simulink model "controller_smp"  (R2021a)
settings: Solver=FixedStepAuto  StartTime=0.0  StopTime=10.0  FixedStep=1/10  RelTol=1e-3
settings Model: EnablePacing=on  PacingRate=3  Creator=DAUIN-Win10  LastModifiedBy=augus
settings DataIOCC: SaveOutput=off  SaveTime=off
settings GRTTargetCC: CombineOutputUpdateFcns=off  MatFileLogging=off

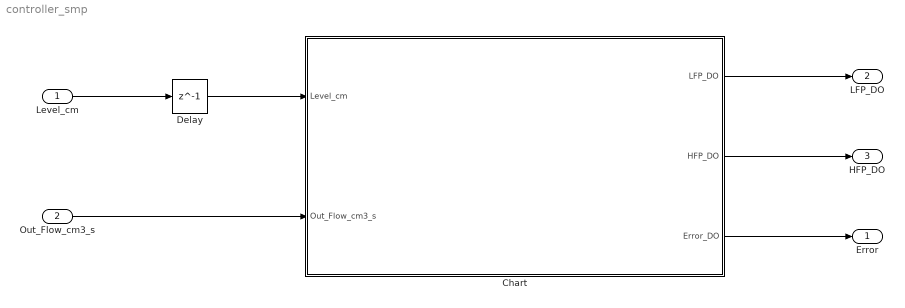
== system controller_smp ==
  Level_cm : Inport  OutDataTypeStr=double
  Out_Flow_cm3_s : Inport  Port=2  OutDataTypeStr=double
  Chart : Stateflow chart  TreatAsAtomicUnit=on
  Delay : Delay  DelayLength=1  InitialCondition=0
  Error : Outport  OutDataTypeStr=uint8
  LFP_DO : Outport  Port=2  OutDataTypeStr=boolean
  HFP_DO : Outport  Port=3  OutDataTypeStr=boolean
  wires:
  Chart/1(LFP_DO) -> LFP_DO/1
  Chart/2(HFP_DO) -> HFP_DO/1
  Chart/3(Error_DO) -> Error/1
  Out_Flow_cm3_s/1 -> Chart/2(Out_Flow_cm3_s)
  Level_cm/1 -> Delay/1
  Delay/1 -> Chart/1(Level_cm)

== stateflow chart controller_smp/Chart ==
  state Control_Logic [parallel]
    settings: executionOrder=1
    state Start
      state High_Flow
        en:
        HFP_DO=1;
        LFP_DO=0;
      state Low_Flow
        en:
        LFP_DO=1;
        HFP_DO=0;
      (default) -> High_Flow
      High_Flow -> Low_Flow : [ Level_cm>155]
      Low_Flow -> High_Flow : [Level_cm<150]
    state Stop
      en:
      LFP_DO=0;
      HFP_DO=0;
    (default) -> Stop
    Start -> Stop : [Level_cm > 180]
    Stop -> Start : [Level_cm<175]
  state Error [parallel]
    settings: executionOrder=2
    state Check_Level [parallel]
      settings: executionOrder=2
      state Error_state
        en:
        Error_DO=1;
      state Normal_state
        en:
        Error_DO=0;
      (default) -> Normal_state
      Normal_state -> Error_state : [Level_cm<=0 || Level_cm >= 200]
    state Check_Pump [parallel]
      settings: executionOrder=1
      state LowFlow_Check
        (default) -> (junction 121)
        (junction 121) -> (junction 122) [order 1] : [(1-Out_Flow_cm3_s/2)>0.75 || (1-Out_Flow_cm3_s/2)<0.5]
        (junction 121) -> (junction 123) [order 2]
        (junction 122) -> (junction 124) : {Error_DO=1;}
        (junction 124) -> (junction 123)
        (junction 123) -> (junction 125)
      state Pump_Off
        (default) -> (junction 97)
        (junction 97) -> (junction 98) [order 1] : [(Out_Flow_cm3_s)/2>0.5 || (Out_Flow_cm3_s)/2<0.25]
        (junction 97) -> (junction 99) [order 2]
        (junction 98) -> (junction 100) : {Error_DO=1;}
        (junction 100) -> (junction 99)
        (junction 99) -> (junction 101)
      state HighFlow_Check
        (default) -> (junction 109)
        (junction 109) -> (junction 110) [order 1] : [(3-Out_Flow_cm3_s/2)>2.75 || (3-Out_Flow_cm3_s/2)<2.5]
        (junction 109) -> (junction 111) [order 2]
        (junction 110) -> (junction 112) : {Error_DO=1;}
        (junction 112) -> (junction 111)
        (junction 111) -> (junction 113)
      (default) -> Pump_Off
      Pump_Off -> LowFlow_Check [order 1] : [LFP_DO==1]
      LowFlow_Check -> Pump_Off : [LFP_DO==0]
      Pump_Off -> HighFlow_Check [order 2] : [HFP_DO==1]
      HighFlow_Check -> Pump_Off : [HFP_DO==0]
    (default) -> Check_Pump
  (default) -> Control_Logic
  data: Level_cm input double size=1; LFP_DO output boolean; HFP_DO output boolean; Error_DO output uint8; Out_Flow_cm3_s input double
